simulink model "KUKA_AdaptiveComposite"  (R2021a)
settings: Solver=FixedStepAuto  StartTime=0.0  StopTime=2  FixedStep=0.001  RelTol=1e-3
InitFcn:
  | Gamma=eye(4)*0.1;
  | K=[1600 1600 1600 1600;80 80 80 80];
  | 
  | Gamma1=diag([20,10,10,15]);
  | K1=[1600 900 900 900;40 40 40 40];
  | 
  | Gamma2=eye(4)*5;
  | K2=[1600 900 900 900; 60 60 60 60];
values from neighbouring files (symbols this model uses):
  m = {0 0 0 0 0}    [DynMatrixCalculator.m]
  N = {zeros(3,1) zeros(3,1) zeros(3,1) zeros(3,1) zeros(3,1)}    [DynMatrixCalculator.m]
undefined symbols (not defined in the file or in its folder): X, Y, Z
libraries: nesl_utility x51, sm_lib x48
(part 1 of 4)
settings Model: Creator=Rahman Ardakanian  LastModifiedBy=hooma
settings SolverCC: AlgebraicLoopSolver=TrustRegion
settings DebuggingCC: SFMachineParentedDataDiag=warning  ArithmeticOperatorsInVariantConditions=warning
settings SFSimCC: CustomCodeUndefinedFunction=UseInterfaceOnly
settings CodeAppCC: StateflowObjectComments=on

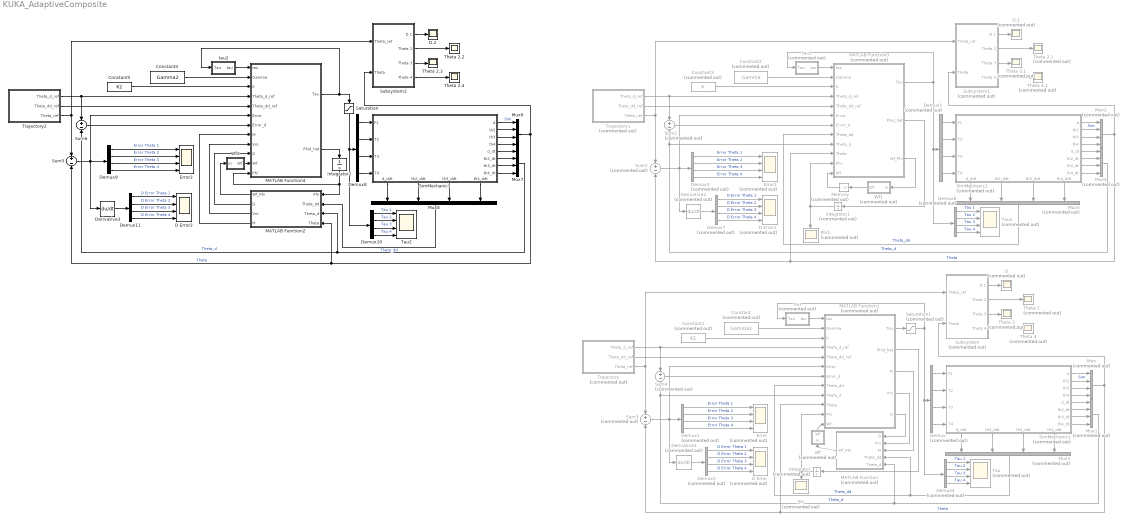
== system KUKA_AdaptiveComposite ==
  Constant : Constant  Commented=on  Value=Gamma1
  Constant1 : Constant  Commented=on  Value=K1
  Constant2 : Constant  Commented=on  Value=Gamma
  Constant3 : Constant  Commented=on  Value=K
  Constant4 : Constant  Value=Gamma2
  Constant5 : Constant  Value=K2
  D : Scope  Commented=on
  D Error : Scope  Commented=on  NumInputPorts=4
  D Error1 : Scope  Commented=on  NumInputPorts=4
  D Error2 : Scope  NumInputPorts=4
  D.1 : Scope  Commented=on
  D.2 : Scope
  Demux{,1..7} (8 alike) : Demux  Commented=on
  Demux{8..11} (4 alike) : Demux
  Derivative1 : Derivative  Commented=on
  Derivative2 : Derivative  Commented=on
  Derivative3 : Derivative
  Error : Scope  Commented=on  NumInputPorts=4
  Error1 : Scope  Commented=on  NumInputPorts=4
  Error2 : Scope  NumInputPorts=4
  Integrator : Integrator  Commented=on  InitialCondition=[17.65,7.84,10.64,8.58,0.186*0.8,0.082*0.8,0.176*0.8,0.166*0.8]
  Integrator1 : Integrator  Commented=on  InitialCondition=[17.65,7.84,10.64,8.58,0.186*0.8,0.082*0.8,0.176*0.8,0.166*0.8]
  Integrator2 : Integrator  InitialCondition=[17.65,7.84,10.64,8.58,0.186*0.8,0.082*0.8,0.176*0.8,0.166*0.8]
  MATLAB Function : MATLAB Function  Commented=on  TreatAsAtomicUnit=on
  MATLAB Function1 : MATLAB Function  Commented=on  TreatAsAtomicUnit=on
  MATLAB Function2 : MATLAB Function  TreatAsAtomicUnit=on
  MATLAB Function3 : MATLAB Function  Commented=on  TreatAsAtomicUnit=on
  MATLAB Function4 : MATLAB Function  TreatAsAtomicUnit=on
  Memory : Memory  Commented=on  InitialCondition=[1,1,1,1]'*0.001
  Mux{,1..5} (6 alike) : Mux  Commented=on
  Mux6 : Mux
  Mux7 : Mux
  Mux8 : Mux
  Phi : Scope  Commented=on
  Phi1 : Scope  Commented=on
  Saturation : Saturate  UpperLimit=[200, 100,100,100]  LowerLimit=-[200, 100,100,100]
  Saturation1 : Saturate  Commented=on  UpperLimit=[200,50,90,30]  LowerLimit=-[200,50,10,10]
  SimMechanic1 : Subsystem  Commented=on
      settings: PortSchema="{\"entries\":[{\"content\":{\"sides\":[{\"content\":{\"connectorIds\":[\"In1\",\"In2\",\"In3\",\"In4\"]},\"type\":\"ConnectorPlacement.EquallySpacedRectSide\",\"uuid\":\"b6277f71-9209-40f9-aaeb-b6c9fa71fb46\"},{\"content\":{\"connectorIds\":[\"Out1\",\"Out2\",\"Out3\",\"Out4\",\"Out5\",\"Out6\",\"Out7\",\"Out8\"],\"side\":\"RIGHT\"},\"type\":\"ConnectorPlacement.EquallySpacedRectSide\",\"uuid\":\"721928da-f16a-424c-b956-77fc0a07fccd\"},{\"content\":{\"connectorIds\":[],\"side\":\"TOP\"},\"type\":\"ConnectorPlacement.EquallySpacedRectSide\",\"uuid\":\"50ddb47d-7b49-4ba3-8344-b30f55dee798\"},{\"content\":{\"connectorIds\":[\"Out9\",\"Out10\",\"Out11\",\"Out12\"],\"side\":\"BOTTOM\"},\"type\":\"ConnectorPlacement.EquallySpacedRectSide\",\"uuid\":\"9af62a72-f078-4531-a2e0-d5b70f194bda\"}]},\"type\":\"ConnectorPlacement.EquallySpacedConnector\",\"uuid\":\"3abc4dda-09b7-4b6a-a507-303450cd9c4c\"}],\"packageUris\":[\"http://schema.mathworks.com/mf0/Connector/R2020b\"],\"version\":\"1.0\"}"
  SimMechanic2 : Subsystem  Commented=on
      settings: PortSchema="{\"entries\":[{\"content\":{\"sides\":[{\"content\":{\"connectorIds\":[\"In1\",\"In2\",\"In3\",\"In4\"]},\"type\":\"ConnectorPlacement.EquallySpacedRectSide\",\"uuid\":\"b6277f71-9209-40f9-aaeb-b6c9fa71fb46\"},{\"content\":{\"connectorIds\":[\"Out1\",\"Out2\",\"Out3\",\"Out4\",\"Out5\",\"Out6\",\"Out7\",\"Out8\"],\"side\":\"RIGHT\"},\"type\":\"ConnectorPlacement.EquallySpacedRectSide\",\"uuid\":\"721928da-f16a-424c-b956-77fc0a07fccd\"},{\"content\":{\"connectorIds\":[],\"side\":\"TOP\"},\"type\":\"ConnectorPlacement.EquallySpacedRectSide\",\"uuid\":\"50ddb47d-7b49-4ba3-8344-b30f55dee798\"},{\"content\":{\"connectorIds\":[\"Out9\",\"Out10\",\"Out11\",\"Out12\"],\"side\":\"BOTTOM\"},\"type\":\"ConnectorPlacement.EquallySpacedRectSide\",\"uuid\":\"9af62a72-f078-4531-a2e0-d5b70f194bda\"}]},\"type\":\"ConnectorPlacement.EquallySpacedConnector\",\"uuid\":\"3abc4dda-09b7-4b6a-a507-303450cd9c4c\"}],\"packageUris\":[\"http://schema.mathworks.com/mf0/Connector/R2020b\"],\"version\":\"1.0\"}"
  SimMechanic3 : Subsystem
      settings: PortSchema="{\"entries\":[{\"content\":{\"sides\":[{\"content\":{\"connectorIds\":[\"In1\",\"In2\",\"In3\",\"In4\"]},\"type\":\"ConnectorPlacement.EquallySpacedRectSide\",\"uuid\":\"b6277f71-9209-40f9-aaeb-b6c9fa71fb46\"},{\"content\":{\"connectorIds\":[\"Out1\",\"Out2\",\"Out3\",\"Out4\",\"Out5\",\"Out6\",\"Out7\",\"Out8\"],\"side\":\"RIGHT\"},\"type\":\"ConnectorPlacement.EquallySpacedRectSide\",\"uuid\":\"721928da-f16a-424c-b956-77fc0a07fccd\"},{\"content\":{\"connectorIds\":[],\"side\":\"TOP\"},\"type\":\"ConnectorPlacement.EquallySpacedRectSide\",\"uuid\":\"50ddb47d-7b49-4ba3-8344-b30f55dee798\"},{\"content\":{\"connectorIds\":[\"Out9\",\"Out10\",\"Out11\",\"Out12\"],\"side\":\"BOTTOM\"},\"type\":\"ConnectorPlacement.EquallySpacedRectSide\",\"uuid\":\"9af62a72-f078-4531-a2e0-d5b70f194bda\"}]},\"type\":\"ConnectorPlacement.EquallySpacedConnector\",\"uuid\":\"3abc4dda-09b7-4b6a-a507-303450cd9c4c\"}],\"packageUris\":[\"http://schema.mathworks.com/mf0/Connector/R2020b\"],\"version\":\"1.0\"}"
  Subsystem : Subsystem  Commented=on
  Subsystem1 : Subsystem  Commented=on
  Subsystem2 : Subsystem
  Sum{1..4} (4 alike) : Sum  Commented=on  Inputs=+|-
  Sum5 : Sum  Inputs=+|-
  Sum6 : Sum  Inputs=+|-
  Tau : Scope  Commented=on  NumInputPorts=4
  Tau1 : Scope  Commented=on  NumInputPorts=4
  Tau2 : Scope  NumInputPorts=4
  Theta 2 : Scope  Commented=on
  Theta 2.1 : Scope  Commented=on
  Theta 2.2 : Scope
  Theta 2.3 : Scope
  Theta 2.4 : Scope
  Theta 3 : Scope  Commented=on
  Theta 3.1 : Scope  Commented=on
  Theta 4 : Scope  Commented=on
  Theta 4.1 : Scope  Commented=on
  Trajectory : Subsystem  Commented=on
  Trajectory1 : Subsystem  Commented=on
  Trajectory2 : Subsystem
  Wf : Subsystem  Commented=on
  Wf1 : Subsystem  Commented=on
  Wf2 : Subsystem
  tau : Subsystem  Commented=on
  tau1 : Subsystem  Commented=on
  tau2 : Subsystem
  wires:
  Wf2/1(Wf) -> MATLAB Function4/11(Wf)
  Demux9/2 -> Error2/2  "Error Theta 2"
  Mux6/1 -> Subsystem2/2(Theta), Sum5/2, MATLAB Function2/4(Theta)  "Theta"
  Derivative3/1 -> Demux11/1
  Mux8/1 -> MATLAB Function2/2(Theta_dd)  "Theta_dd"
  SimMechanic3/1(d) -> Mux6/1  "Sim"
  SimMechanic3/2(th2) -> Mux6/2
  SimMechanic3/4(th4) -> Mux6/4
  Trajectory2/3(Theta_ref) -> Sum5/1, Subsystem2/1(Theta_ref)
  Demux8/3 -> SimMechanic3/3(T3)
  MATLAB Function2/1(Wf_Phi) -> Wf2/1(in)
  SimMechanic3/7(th3_dt) -> Mux7/3
  SimMechanic3/12(th4_ddt) -> Mux8/4
  Demux9/1 -> Error2/1  "Error Theta 1"
  SimMechanic3/3(th3) -> Mux6/3
  Demux10/2 -> Tau2/2  "Tau 2"
  Constant5/1 -> MATLAB Function4/3(K)
  Demux8/1 -> SimMechanic3/1(F1)
  SimMechanic3/8(th4_dt) -> Mux7/4
  SimMechanic3/5(d_dt) -> Mux7/1
  Demux9/3 -> Error2/3  "Error Theta 3"
  SimMechanic3/10(th2_ddt) -> Mux8/2
  Demux11/3 -> D Error2/3  "D Error Theta 3"
  SimMechanic3/6(th2_dt) -> Mux7/2
  SimMechanic3/11(th3_ddt) -> Mux8/3
  Demux11/4 -> D Error2/4  "D Error Theta 4"
  Trajectory2/1(Theta_d_ref) -> Sum6/1, MATLAB Function4/4(Theta_d_ref)
  Mux7/1 -> Sum6/2, MATLAB Function2/3(Theta_d)  "Theta_d"
  Trajectory2/2(Theta_dd_ref) -> MATLAB Function4/5(Theta_dd_ref)
  Demux10/3 -> Tau2/3  "Tau 3"
  Subsystem2/1(D 1) -> D.2/1
  Sum6/1 -> MATLAB Function4/7(Error_d)
  Demux11/2 -> D Error2/2  "D Error Theta 2"
  Subsystem2/4(Theta 4) -> Theta 2.4/1
  SimMechanic3/9(d_ddt) -> Mux8/1
  Demux10/1 -> Tau2/1  "Tau 1"
  Constant4/1 -> MATLAB Function4/2(Gamma)
  Subsystem2/2(Theta 2) -> Theta 2.2/1
  Subsystem2/3(Theta 3) -> Theta 2.3/1
  Demux10/4 -> Tau2/4  "Tau 4"
  Sum5/1 -> Derivative3/1, MATLAB Function4/6(Error), Demux9/1
  Demux8/4 -> SimMechanic3/4(T4)
  Demux11/1 -> D Error2/1  "D Error Theta 1"
  tau2/1(tau) -> MATLAB Function4/1(tau)
  Demux9/4 -> Error2/4  "Error Theta 4"
  Demux8/2 -> SimMechanic3/2(T2)
  MATLAB Function2/2(G) -> MATLAB Function4/10(G)
  MATLAB Function2/3(Vm) -> MATLAB Function4/9(Vm)
  MATLAB Function2/4(M) -> MATLAB Function4/8(M)
  MATLAB Function4/2(Phid_hat) -> Integrator2/1
  Integrator2/1 -> MATLAB Function2/1(Phi), MATLAB Function4/12(Phi)
  Saturation/1 -> Demux10/1, Demux8/1
  MATLAB Function4/1(Tau) -> tau2/1(Tau), Saturation/1
  Demux3/4 -> Error1/4  "Error Theta 4"
  Demux1/1 -> Error/1  "Error Theta 1"
  SimMechanic1/7(th3_dt) -> Mux1/3
  Trajectory/1(Theta_d_ref) -> Sum4/1, MATLAB Function1/4(Theta_d_ref)
  Demux5/4 -> D Error/4  "D Error Theta 4"
  Sum1/1 -> Derivative2/1, Demux3/1, MATLAB Function3/6(Error)
  SimMechanic2/7(th3_dt) -> Mux4/3
  SimMechanic1/12(th4_ddt) -> Mux3/4
  Demux/2 -> SimMechanic1/2(T2)
  Constant1/1 -> MATLAB Function1/3(K)
  Subsystem1/4(Theta 4) -> Theta 4.1/1
  Derivative1/1 -> Demux5/1
  SimMechanic1/6(th2_dt) -> Mux1/2
  SimMechanic2/4(th4) -> Mux2/4
  Demux/3 -> SimMechanic1/3(T3)
  Constant2/1 -> MATLAB Function3/2(Gamma)
  SimMechanic1/5(d_dt) -> Mux1/1
  Demux5/1 -> D Error/1  "D Error Theta 1"
  MATLAB Function1/4(Vm) -> MATLAB Function/2(Vm)
  Demux3/2 -> Error1/2  "Error Theta 2"
  tau/1(tau) -> MATLAB Function1/1(tau)
  MATLAB Function3/3(Wf_Phi) -> Wf1/1(in)
  Demux2/3 -> SimMechanic2/3(T3)
  SimMechanic1/1(d) -> Mux/1  "Sim"
  Integrator1/1 -> Phi1/1, MATLAB Function3/11(Phi)
  Demux6/2 -> Tau1/2  "Tau 2"
  Wf1/1(Wf) -> Memory/1
  Demux/1 -> SimMechanic1/1(F1)
  Subsystem/4(Theta 4) -> Theta 4/1
  SimMechanic1/11(th3_ddt) -> Mux3/3
  Saturation1/1 -> tau/1(Tau), Demux4/1, Demux/1
  MATLAB Function1/5(G) -> MATLAB Function/1(G)
  SimMechanic1/3(th3) -> Mux/3
  Demux3/1 -> Error1/1  "Error Theta 1"
  SimMechanic2/12(th4_ddt) -> Mux5/4
  SimMechanic2/3(th3) -> Mux2/3
  Memory/1 -> MATLAB Function3/12(Wf)
  Demux/4 -> SimMechanic1/4(T4)
  SimMechanic2/5(d_dt) -> Mux4/1
  Demux5/2 -> D Error/2  "D Error Theta 2"
  Demux4/3 -> Tau/3  "Tau 3"
  Subsystem/2(Theta 2) -> Theta 2/1
  Demux4/4 -> Tau/4  "Tau 4"
  Demux4/1 -> Tau/1  "Tau 1"
  Mux/1 -> Subsystem/2(Theta), MATLAB Function1/10(Theta), Sum3/2  "Theta"
  Demux1/3 -> Error/3  "Error Theta 3"
  Demux2/2 -> SimMechanic2/2(T2)
  SimMechanic1/2(th2) -> Mux/2
  Mux5/1 -> MATLAB Function3/8(Theta_dd)  "Theta_dd"
  Demux5/3 -> D Error/3  "D Error Theta 3"
  Demux6/1 -> Tau1/1  "Tau 1"
  Demux2/4 -> SimMechanic2/4(T4)
  Demux4/2 -> Tau/2  "Tau 2"
  SimMechanic1/8(th4_dt) -> Mux1/4
  SimMechanic1/10(th2_ddt) -> Mux3/2
  Subsystem/1(D 1) -> D/1
  Integrator/1 -> MATLAB Function1/11(Phi), Phi/1
  SimMechanic1/9(d_ddt) -> Mux3/1
  Mux3/1 -> MATLAB Function1/8(Theta_dd), MATLAB Function/4(Theta_dd)  "Theta_dd"
  Mux1/1 -> MATLAB Function/5(Theta_d), Sum4/2, MATLAB Function1/9(Theta_d)  "Theta_d"
  Sum4/1 -> MATLAB Function1/7(Error_d)
  Subsystem1/2(Theta 2) -> Theta 2.1/1
  Demux6/3 -> Tau1/3  "Tau 3"
  SimMechanic2/2(th2) -> Mux2/2
  Constant3/1 -> MATLAB Function3/3(K)
  Demux7/1 -> D Error1/1  "D Error Theta 1"
  SimMechanic1/4(th4) -> Mux/4
  Subsystem1/1(D 1) -> D.1/1
  Subsystem/3(Theta 3) -> Theta 3/1
  Demux6/4 -> Tau1/4  "Tau 4"
  Constant/1 -> MATLAB Function1/2(Gamma)
  Wf/1(Wf) -> MATLAB Function1/12(Wf)
  Demux1/2 -> Error/2  "Error Theta 2"
  MATLAB Function/1(Wf_Phi) -> Wf/1(in)
  SimMechanic2/1(d) -> Mux2/1  "Sim"
  MATLAB Function1/3(M) -> MATLAB Function/3(M)
  SimMechanic2/8(th4_dt) -> Mux4/4
  Trajectory/2(Theta_dd_ref) -> MATLAB Function1/5(Theta_dd_ref)
  SimMechanic2/9(d_ddt) -> Mux5/1
  Demux7/2 -> D Error1/2  "D Error Theta 2"
  MATLAB Function3/1(Tau) -> tau1/1(Tau), Demux6/1, Demux2/1
  MATLAB Function1/2(Phid_hat) -> Integrator/1
  SimMechanic2/11(th3_ddt) -> Mux5/3
  SimMechanic2/6(th2_dt) -> Mux4/2
  Derivative2/1 -> Demux7/1
  Mux2/1 -> Subsystem1/2(Theta), MATLAB Function3/10(Theta), Sum1/2  "Theta"
  Mux4/1 -> Sum2/2, MATLAB Function3/9(Theta_d)  "Theta_d"
  Sum3/1 -> Derivative1/1, Demux1/1, MATLAB Function1/6(Error)
  tau1/1(tau) -> MATLAB Function3/1(tau)
  MATLAB Function1/1(Tau) -> Saturation1/1
  MATLAB Function3/2(Phid_hat) -> Integrator1/1
  Demux3/3 -> Error1/3  "Error Theta 3"
  Demux2/1 -> SimMechanic2/1(F1)
  Trajectory1/2(Theta_dd_ref) -> MATLAB Function3/5(Theta_dd_ref)
  Trajectory/3(Theta_ref) -> Sum3/1, Subsystem/1(Theta_ref)
  Demux1/4 -> Error/4  "Error Theta 4"
  Trajectory1/1(Theta_d_ref) -> Sum2/1, MATLAB Function3/4(Theta_d_ref)
  SimMechanic2/10(th2_ddt) -> Mux5/2
  Demux7/4 -> D Error1/4  "D Error Theta 4"
  Sum2/1 -> MATLAB Function3/7(Error_d)
  Trajectory1/3(Theta_ref) -> Sum1/1, Subsystem1/1(Theta_ref)
  Subsystem1/3(Theta 3) -> Theta 3.1/1
  Demux7/3 -> D Error1/3  "D Error Theta 3"

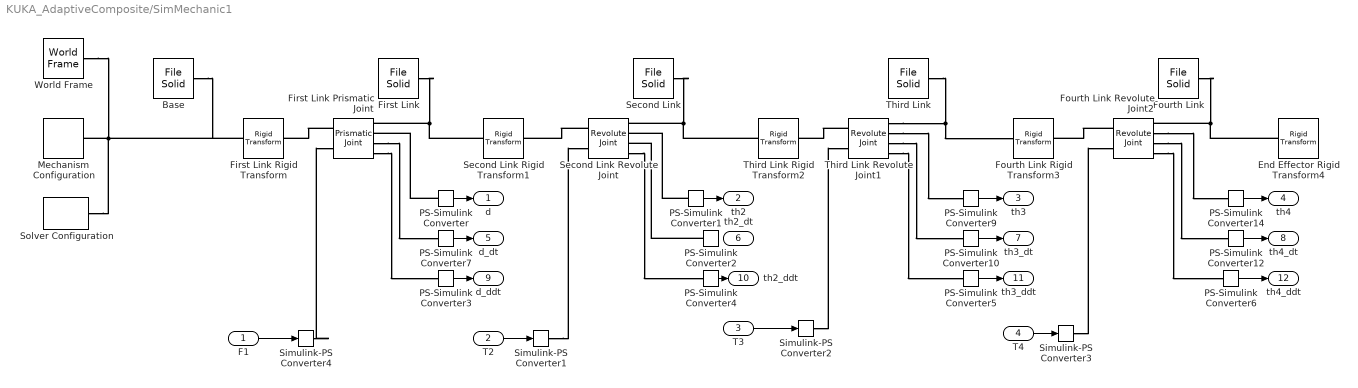
== system KUKA_AdaptiveComposite/SimMechanic1 ==
  F1 : Inport
  T2 : Inport  Port=2
  T3 : Inport  Port=3
  T4 : Inport  Port=4
  Base : sm_lib/Body Elements/File Solid  ExtGeomFileName=L0.STL  UnitType=Custom  ExtGeomFileUnits=mm  StepReaderType=HEX  ExportConvexHullGeometry=off  InertiaType=Custom  Mass=40.117  MassUnits=kg  CenterOfMass=[0 -0.033 0]  CenterOfMassUnits=m  MomentsOfInertia=[13.366 13.428 0.066]  MomentsOfInertiaUnits=kg*m^2  ProductsOfInertia=[0 0 0]  ProductsOfInertiaUnits=kg*m^2  BasedOnType=Density  Density=1000  DensityUnits=kg/m^3  DoExposeReferenceFrame=on  SerializedFrames=<Frames/>  GraphicType=FromGeometry  MarkerShape=Sphere  MarkerSize=10  GraphicVisPropType=SimpleVisualProperties  GraphicDiffuseColor=[0.5 0.5 0.5]  GraphicSpecularColor=[0.5 0.5 0.5 1.0]  GraphicAmbientColor=[0.15 0.15 0.15 1.0]  GraphicEmissiveColor=[0.0 0.0 0.0 1.0]  GraphicShininess=75  GraphicOpacity=1.0
  End Effector Rigid Transform4 : sm_lib/Frames and Transforms/Rigid Transform  TranslationMethod=Cartesian  TranslationStandardOffset=0  TranslationLengthUnit=mm  TranslationStandardAxis=+Z  TranslationCartesianOffset=[382.6 20 0]  TranslationROffset=0  TranslationROffsetUnits=m  TranslationZOffset=0  TranslationZOffsetUnits=m  TranslationThetaOffset=0  TranslationThetaOffsetUnits=deg  RotationMethod=AlignedAxes  RotationAngleUnits=deg  RotationStandardAxis=+Z  RotationAngle=0.0  RotationArbitraryAxis=[0 0 1]  FollAlignAxisA=+X  BaseAlignAxisA=+X  FollAlignAxisB=+Y  BaseAlignAxisB=+Y  RotationSequenceAxes=FollowerAxes  RotationSequence=XYX  RotationSequenceAngles=[0 0 0]  RotationSequenceAnglesUnits=deg  RotationMatrix=[1 0 0; 0 1 0; 0 0 1]
  First Link : sm_lib/Body Elements/File Solid  ExtGeomFileName=L1.STL  UnitType=Custom  ExtGeomFileUnits=mm  StepReaderType=HEX  ExportConvexHullGeometry=off  InertiaType=Custom  Mass=22.064  MassUnits=kg  CenterOfMass=[-0.031 0.094 0]  CenterOfMassUnits=m  MomentsOfInertia=[0.134 0.165 0.186]  MomentsOfInertiaUnits=kg*m^2  ProductsOfInertia=[0 0.001 -0.012]  ProductsOfInertiaUnits=kg*m^2  BasedOnType=Density  Density=1000  DensityUnits=kg/m^3  DoExposeReferenceFrame=on  SerializedFrames=<Frames/>  GraphicType=FromGeometry  MarkerShape=Sphere  MarkerSize=10  GraphicVisPropType=SimpleVisualProperties  GraphicDiffuseColor=[0.5 0.5 0.5]  GraphicSpecularColor=[0.5 0.5 0.5 1.0]  GraphicAmbientColor=[0.15 0.15 0.15 1.0]  GraphicEmissiveColor=[0.0 0.0 0.0 1.0]  GraphicShininess=75  GraphicOpacity=1.0
  First Link Prismatic Joint : sm_lib/Joints/Prismatic Joint  JointMode=Normal  SenseConstraintForce=off  SenseConstraintForceX=off  SenseConstraintForceY=off  SenseConstraintForceZ=off  SenseConstraintTorque=off  SenseConstraintTorqueX=off  SenseConstraintTorqueY=off  SenseConstraintTorqueZ=off  SenseTotalForce=off  SenseTotalForceX=off  SenseTotalForceY=off  SenseTotalForceZ=off  SenseTotalTorque=off  SenseTotalTorqueX=off  SenseTotalTorqueY=off  SenseTotalTorqueZ=off  CompositeWrenchDir=FollowerOnBase  CompositeWrenchFrame=BaseFrame  EquilibriumPosition=0  EquilibriumPositionUnits=m  SpringStiffness=0  SpringStiffnessUnits=N/m  DampingCoefficient=0  DampingCoefficientUnits=N/(m/s)  TorqueActuationMode=InputTorque  MotionActuationMode=ComputedMotion  SensePosition=on  SenseVelocity=on  SenseAcceleration=on  SenseTorqueForce=off  SenseLowerLimitTorqueForce=off  SenseUpperLimitTorqueForce=off  LowerLimitSpecify=off  LowerLimitBound=-1  LowerLimitBoundUnits=m  LowerLimitStiffness=1e6  LowerLimitStiffnessUnits=N/m  LowerLimitDamping=1e3  LowerLimitDampingUnits=N/(m/s)  LowerLimitTransitionRegionWidth=1e-4  LowerLimitTransitionRegionWidthUnits=m  UpperLimitSpecify=off  UpperLimitBound=1  UpperLimitBoundUnits=m  UpperLimitStiffness=1e6  UpperLimitStiffnessUnits=N/m  UpperLimitDamping=1e3  UpperLimitDampingUnits=N/(m/s)  UpperLimitTransitionRegionWidth=1e-4  UpperLimitTransitionRegionWidthUnits=m  PositionTargetSpecify=off  PositionTargetPriority=High  PositionTargetValue=0  PositionTargetValueUnits=m  VelocityTargetSpecify=off  VelocityTargetPriority=High  VelocityTargetValue=0  VelocityTargetValueUnits=m/s
  First Link Rigid Transform : sm_lib/Frames and Transforms/Rigid Transform  TranslationMethod=Cartesian  TranslationStandardOffset=0  TranslationLengthUnit=mm  TranslationStandardAxis=+Z  TranslationCartesianOffset=[0 0 0]  TranslationROffset=0  TranslationROffsetUnits=m  TranslationZOffset=0  TranslationZOffsetUnits=m  TranslationThetaOffset=0  TranslationThetaOffsetUnits=deg  RotationMethod=AlignedAxes  RotationAngleUnits=deg  RotationStandardAxis=+Z  RotationAngle=0.0  RotationArbitraryAxis=[0 0 1]  FollAlignAxisA=+X  BaseAlignAxisA=+X  FollAlignAxisB=+Y  BaseAlignAxisB=+Y  RotationSequenceAxes=FollowerAxes  RotationSequence=XYX  RotationSequenceAngles=[0 0 0]  RotationSequenceAnglesUnits=deg  RotationMatrix=[1 0 0; 0 1 0; 0 0 1]
  Fourth Link : sm_lib/Body Elements/File Solid  ExtGeomFileName=L4.STL  UnitType=Custom  ExtGeomFileUnits=mm  StepReaderType=HEX  ExportConvexHullGeometry=off  InertiaType=Custom  Mass=10.723  MassUnits=kg  CenterOfMass=[0.143 0.015 -0.001]  CenterOfMassUnits=m  MomentsOfInertia=[0.018 0.166 0.164]  MomentsOfInertiaUnits=kg*m^2  ProductsOfInertia=[0 -0.001 0.009]  ProductsOfInertiaUnits=kg*m^2  BasedOnType=Density  Density=1000  DensityUnits=kg/m^3  DoExposeReferenceFrame=on  SerializedFrames=<Frames/>  GraphicType=FromGeometry  MarkerShape=Sphere  MarkerSize=10  GraphicVisPropType=SimpleVisualProperties  GraphicDiffuseColor=[0.5 0.5 0.5]  GraphicSpecularColor=[0.5 0.5 0.5 1.0]  GraphicAmbientColor=[0.15 0.15 0.15 1.0]  GraphicEmissiveColor=[0.0 0.0 0.0 1.0]  GraphicShininess=75  GraphicOpacity=1.0
  Fourth Link Revolute Joint2 : sm_lib/Joints/Revolute Joint  JointMode=Normal  SenseConstraintForce=off  SenseConstraintForceX=off  SenseConstraintForceY=off  SenseConstraintForceZ=off  SenseConstraintTorque=off  SenseConstraintTorqueX=off  SenseConstraintTorqueY=off  SenseConstraintTorqueZ=off  SenseTotalForce=off  SenseTotalForceX=off  SenseTotalForceY=off  SenseTotalForceZ=off  SenseTotalTorque=off  SenseTotalTorqueX=off  SenseTotalTorqueY=off  SenseTotalTorqueZ=off  CompositeWrenchDir=FollowerOnBase  CompositeWrenchFrame=BaseFrame  EquilibriumPosition=0  EquilibriumPositionUnits=deg  SpringStiffness=0  SpringStiffnessUnits=N*m/deg  DampingCoefficient=0  DampingCoefficientUnits=N*m/(deg/s)  TorqueActuationMode=InputTorque  MotionActuationMode=ComputedMotion  SensePosition=on  SenseVelocity=on  SenseAcceleration=on  SenseTorqueForce=off  SenseLowerLimitTorqueForce=off  SenseUpperLimitTorqueForce=off  LowerLimitSpecify=off  LowerLimitBound=-90  LowerLimitBoundUnits=deg  LowerLimitStiffness=1e4  LowerLimitStiffnessUnits=N*m/deg  LowerLimitDamping=10  LowerLimitDampingUnits=N*m/(deg/s)  LowerLimitTransitionRegionWidth=0.1  LowerLimitTransitionRegionWidthUnits=deg  UpperLimitSpecify=off  UpperLimitBound=90  UpperLimitBoundUnits=deg  UpperLimitStiffness=1e4  UpperLimitStiffnessUnits=N*m/deg  UpperLimitDamping=10  UpperLimitDampingUnits=N*m/(deg/s)  UpperLimitTransitionRegionWidth=0.1  UpperLimitTransitionRegionWidthUnits=deg  PositionTargetSpecify=off  PositionTargetPriority=High  PositionTargetValue=0  PositionTargetValueUnits=deg  VelocityTargetSpecify=off  VelocityTargetPriority=High  VelocityTargetValue=0  VelocityTargetValueUnits=deg/s
  Fourth Link Rigid Transform3 : sm_lib/Frames and Transforms/Rigid Transform  TranslationMethod=Cartesian  TranslationStandardOffset=0  TranslationLengthUnit=mm  TranslationStandardAxis=+Z  TranslationCartesianOffset=[290 0 0]  TranslationROffset=0  TranslationROffsetUnits=m  TranslationZOffset=0  TranslationZOffsetUnits=m  TranslationThetaOffset=0  TranslationThetaOffsetUnits=deg  RotationMethod=AlignedAxes  RotationAngleUnits=deg  RotationStandardAxis=+Z  RotationAngle=0.0  RotationArbitraryAxis=[0 0 1]  FollAlignAxisA=+X  BaseAlignAxisA=-Y  FollAlignAxisB=+Z  BaseAlignAxisB=+Z  RotationSequenceAxes=FollowerAxes  RotationSequence=XYX  RotationSequenceAngles=[0 0 0]  RotationSequenceAnglesUnits=deg  RotationMatrix=[1 0 0; 0 1 0; 0 0 1]
  Mechanism Configuration : sm_lib/Utilities/Mechanism Configuration  UniformGravity=Constant  GravityVector=[0 -9.80665 0]  GravityVectorUnits=m/s^2  GravityUnits=m/s^2  LinearizationDelta=0.001  JointModeTransitionNonlinearIterations=2
  PS-Simulink Converter : nesl_utility/PS-Simulink Converter  PhysicalDomain=network_engine_domain  SubClassName=ps_output  LeftPortType=input  RightPortType=output  PseudoPeriodic=off  Frequencies=[]  Unit=m  AffineConversion=off
      settings: SourceProductBaseCode=PW,SS
  PS-Simulink Converter1 : nesl_utility/PS-Simulink Converter  PhysicalDomain=network_engine_domain  SubClassName=ps_output  LeftPortType=input  RightPortType=output  PseudoPeriodic=off  Frequencies=[]  Unit=rad  AffineConversion=off
      settings: SourceProductBaseCode=PW,SS
  PS-Simulink Converter10 : nesl_utility/PS-Simulink Converter  PhysicalDomain=network_engine_domain  SubClassName=ps_output  LeftPortType=input  RightPortType=output  PseudoPeriodic=off  Frequencies=[]  Unit=rad/s  AffineConversion=off
      settings: SourceProductBaseCode=PW,SS
  PS-Simulink Converter12 : nesl_utility/PS-Simulink Converter  PhysicalDomain=network_engine_domain  SubClassName=ps_output  LeftPortType=input  RightPortType=output  PseudoPeriodic=off  Frequencies=[]  Unit=rad/s  AffineConversion=off
      settings: SourceProductBaseCode=PW,SS
  PS-Simulink Converter14 : nesl_utility/PS-Simulink Converter  PhysicalDomain=network_engine_domain  SubClassName=ps_output  LeftPortType=input  RightPortType=output  PseudoPeriodic=off  Frequencies=[]  Unit=rad  AffineConversion=off
      settings: SourceProductBaseCode=PW,SS
  PS-Simulink Converter2 : nesl_utility/PS-Simulink Converter  PhysicalDomain=network_engine_domain  SubClassName=ps_output  LeftPortType=input  RightPortType=output  PseudoPeriodic=off  Frequencies=[]  Unit=rad/s  AffineConversion=off
      settings: SourceProductBaseCode=PW,SS
  PS-Simulink Converter3 : nesl_utility/PS-Simulink Converter  PhysicalDomain=network_engine_domain  SubClassName=ps_output  LeftPortType=input  RightPortType=output  PseudoPeriodic=off  Frequencies=[]  Unit=m/s^2  AffineConversion=off
      settings: SourceProductBaseCode=PW,SS
  PS-Simulink Converter4 : nesl_utility/PS-Simulink Converter  PhysicalDomain=network_engine_domain  SubClassName=ps_output  LeftPortType=input  RightPortType=output  PseudoPeriodic=off  Frequencies=[]  Unit=rad/s^2  AffineConversion=off
      settings: SourceProductBaseCode=PW,SS
  PS-Simulink Converter5 : nesl_utility/PS-Simulink Converter  PhysicalDomain=network_engine_domain  SubClassName=ps_output  LeftPortType=input  RightPortType=output  PseudoPeriodic=off  Frequencies=[]  Unit=rad/s^2  AffineConversion=off
      settings: SourceProductBaseCode=PW,SS
  PS-Simulink Converter6 : nesl_utility/PS-Simulink Converter  PhysicalDomain=network_engine_domain  SubClassName=ps_output  LeftPortType=input  RightPortType=output  PseudoPeriodic=off  Frequencies=[]  Unit=rad/s^2  AffineConversion=off
      settings: SourceProductBaseCode=PW,SS
  PS-Simulink Converter7 : nesl_utility/PS-Simulink Converter  PhysicalDomain=network_engine_domain  SubClassName=ps_output  LeftPortType=input  RightPortType=output  PseudoPeriodic=off  Frequencies=[]  Unit=m/s  AffineConversion=off
      settings: SourceProductBaseCode=PW,SS
  PS-Simulink Converter9 : nesl_utility/PS-Simulink Converter  PhysicalDomain=network_engine_domain  SubClassName=ps_output  LeftPortType=input  RightPortType=output  PseudoPeriodic=off  Frequencies=[]  Unit=rad  AffineConversion=off
      settings: SourceProductBaseCode=PW,SS
  Second Link : sm_lib/Body Elements/File Solid  ExtGeomFileName=L2.STL  UnitType=Custom  ExtGeomFileUnits=mm  StepReaderType=HEX  ExportConvexHullGeometry=off  InertiaType=Custom  Mass=9.805  MassUnits=kg  CenterOfMass=[-0.005 -0.001 0.082]  CenterOfMassUnits=m  MomentsOfInertia=[0.082 0.053 0.058]  MomentsOfInertiaUnits=kg*m^2  ProductsOfInertia=[-0.001 0 0]  ProductsOfInertiaUnits=kg*m^2  BasedOnType=Density  Density=1000  DensityUnits=kg/m^3  DoExposeReferenceFrame=on  SerializedFrames=<Frames/>  GraphicType=FromGeometry  MarkerShape=Sphere  MarkerSize=10  GraphicVisPropType=SimpleVisualProperties  GraphicDiffuseColor=[0.5 0.5 0.5]  GraphicSpecularColor=[0.5 0.5 0.5 1.0]  GraphicAmbientColor=[0.15 0.15 0.15 1.0]  GraphicEmissiveColor=[0.0 0.0 0.0 1.0]  GraphicShininess=75  GraphicOpacity=1.0
  Second Link Revolute Joint : sm_lib/Joints/Revolute Joint  JointMode=Normal  SenseConstraintForce=off  SenseConstraintForceX=off  SenseConstraintForceY=off  SenseConstraintForceZ=off  SenseConstraintTorque=off  SenseConstraintTorqueX=off  SenseConstraintTorqueY=off  SenseConstraintTorqueZ=off  SenseTotalForce=off  SenseTotalForceX=off  SenseTotalForceY=off  SenseTotalForceZ=off  SenseTotalTorque=off  SenseTotalTorqueX=off  SenseTotalTorqueY=off  SenseTotalTorqueZ=off  CompositeWrenchDir=FollowerOnBase  CompositeWrenchFrame=BaseFrame  EquilibriumPosition=0  EquilibriumPositionUnits=deg  SpringStiffness=0  SpringStiffnessUnits=N*m/deg  DampingCoefficient=0  DampingCoefficientUnits=N*m/(deg/s)  TorqueActuationMode=InputTorque  MotionActuationMode=ComputedMotion  SensePosition=on  SenseVelocity=on  SenseAcceleration=on  SenseTorqueForce=off  SenseLowerLimitTorqueForce=off  SenseUpperLimitTorqueForce=off  LowerLimitSpecify=off  LowerLimitBound=-90  LowerLimitBoundUnits=deg  LowerLimitStiffness=1e4  LowerLimitStiffnessUnits=N*m/deg  LowerLimitDamping=10  LowerLimitDampingUnits=N*m/(deg/s)  LowerLimitTransitionRegionWidth=0.1  LowerLimitTransitionRegionWidthUnits=deg  UpperLimitSpecify=off  UpperLimitBound=90  UpperLimitBoundUnits=deg  UpperLimitStiffness=1e4  UpperLimitStiffnessUnits=N*m/deg  UpperLimitDamping=10  UpperLimitDampingUnits=N*m/(deg/s)  UpperLimitTransitionRegionWidth=0.1  UpperLimitTransitionRegionWidthUnits=deg  PositionTargetSpecify=off  PositionTargetPriority=High  PositionTargetValue=0  PositionTargetValueUnits=deg  VelocityTargetSpecify=off  VelocityTargetPriority=High  VelocityTargetValue=0  VelocityTargetValueUnits=deg/s
  Second Link Rigid Transform1 : sm_lib/Frames and Transforms/Rigid Transform  TranslationMethod=Cartesian  TranslationStandardOffset=0  TranslationLengthUnit=mm  TranslationStandardAxis=+Z  TranslationCartesianOffset=[0 197 0]  TranslationROffset=0  TranslationROffsetUnits=m  TranslationZOffset=0  TranslationZOffsetUnits=m  TranslationThetaOffset=0  TranslationThetaOffsetUnits=deg  RotationMethod=AlignedAxes  RotationAngleUnits=deg  RotationStandardAxis=+Z  RotationAngle=0.0  RotationArbitraryAxis=[0 0 1]  FollAlignAxisA=+X  BaseAlignAxisA=+X  FollAlignAxisB=+Y  BaseAlignAxisB=-Z  RotationSequenceAxes=FollowerAxes  RotationSequence=XYX  RotationSequenceAngles=[0 0 0]  RotationSequenceAnglesUnits=deg  RotationMatrix=[1 0 0; 0 1 0; 0 0 1]
  Simulink-PS Converter{1..4} (4 alike) : nesl_utility/Simulink-PS Converter  PhysicalDomain=network_engine_domain  SubClassName=ps_input  LeftPortType=input  RightPortType=output  PseudoPeriodic=off  Frequencies=[]  NoiseDistribution=none  NoiseParameters=[]  Unit=1  AffineConversion=off  FilteringAndDerivatives=provide  SimscapeFilterOrder=1  InputFilterTimeConstant=0.001  UdotUserProvided=0
      settings: SourceProductBaseCode=PW,SS
  Solver Configuration : nesl_utility/Solver Configuration  PhysicalDomain=network_engine_domain  SubClassName=solver  LeftPortType=input  RightPortType=generic  Tones=[]  Harmonics=[]  SimulateNoise=off  Profile=off  UseLocalSampling=off  EnableSwitchedLinearOptims=on  FrequencyDomain=off  UseCCode=off  RelTol=0.001  AbsTol=1e-06  MinStep=1e-09  ToWorkspace=off  RevertToSquareIcSolve=off  NumHomotopyIterations=100  PhasorMode=off  PhasorModeNumHarmonics=1  DoDC=off  ResidualTolerance=1e-09  UseLocalSolver=off  LocalSolverChoice=NE_BACKWARD_EULER_ADVANCER  LocalSolverSampleTime=0.001  DoFixedCost=off  MaxNonlinIter=3  MaxModeIter=2  ComputeImpulses=off  ImpulseIterations=2  LinearAlgebra=Sparse  EquationFormulation=NE_TIME_EF  DelaysMemoryBudget=1024  AutomaticFiltering=on  FilteringTimeConstant=0.001  PartitionStorageMethod=AS_NEEDED  PartitionMemoryBudget=1024  PartitionMethod=FAST
      settings: SourceProductBaseCode=PW,SS
  Third Link : sm_lib/Body Elements/File Solid  ExtGeomFileName=L3.STL  UnitType=Custom  ExtGeomFileUnits=mm  StepReaderType=HEX  ExportConvexHullGeometry=off  InertiaType=Custom  Mass=13.302  MassUnits=kg  CenterOfMass=[0.118 0.011 -0.001]  CenterOfMassUnits=m  MomentsOfInertia=[0.048 0.176 0.154]  MomentsOfInertiaUnits=kg*m^2  ProductsOfInertia=[0 0.002 0.003]  ProductsOfInertiaUnits=kg*m^2  BasedOnType=Density  Density=1000  DensityUnits=kg/m^3  DoExposeReferenceFrame=on  SerializedFrames=<Frames/>  GraphicType=FromGeometry  MarkerShape=Sphere  MarkerSize=10  GraphicVisPropType=SimpleVisualProperties  GraphicDiffuseColor=[0.5 0.5 0.5]  GraphicSpecularColor=[0.5 0.5 0.5 1.0]  GraphicAmbientColor=[0.15 0.15 0.15 1.0]  GraphicEmissiveColor=[0.0 0.0 0.0 1.0]  GraphicShininess=75  GraphicOpacity=1.0
  Third Link Revolute Joint1 : sm_lib/Joints/Revolute Joint  JointMode=Normal  SenseConstraintForce=off  SenseConstraintForceX=off  SenseConstraintForceY=off  SenseConstraintForceZ=off  SenseConstraintTorque=off  SenseConstraintTorqueX=off  SenseConstraintTorqueY=off  SenseConstraintTorqueZ=off  SenseTotalForce=off  SenseTotalForceX=off  SenseTotalForceY=off  SenseTotalForceZ=off  SenseTotalTorque=off  SenseTotalTorqueX=off  SenseTotalTorqueY=off  SenseTotalTorqueZ=off  CompositeWrenchDir=FollowerOnBase  CompositeWrenchFrame=BaseFrame  EquilibriumPosition=0  EquilibriumPositionUnits=deg  SpringStiffness=0  SpringStiffnessUnits=N*m/deg  DampingCoefficient=0  DampingCoefficientUnits=N*m/(deg/s)  TorqueActuationMode=InputTorque  MotionActuationMode=ComputedMotion  SensePosition=on  SenseVelocity=on  SenseAcceleration=on  SenseTorqueForce=off  SenseLowerLimitTorqueForce=off  SenseUpperLimitTorqueForce=off  LowerLimitSpecify=off  LowerLimitBound=-90  LowerLimitBoundUnits=deg  LowerLimitStiffness=1e4  LowerLimitStiffnessUnits=N*m/deg  LowerLimitDamping=10  LowerLimitDampingUnits=N*m/(deg/s)  LowerLimitTransitionRegionWidth=0.1  LowerLimitTransitionRegionWidthUnits=deg  UpperLimitSpecify=off  UpperLimitBound=90  UpperLimitBoundUnits=deg  UpperLimitStiffness=1e4  UpperLimitStiffnessUnits=N*m/deg  UpperLimitDamping=10  UpperLimitDampingUnits=N*m/(deg/s)  UpperLimitTransitionRegionWidth=0.1  UpperLimitTransitionRegionWidthUnits=deg  PositionTargetSpecify=off  PositionTargetPriority=High  PositionTargetValue=0  PositionTargetValueUnits=deg  VelocityTargetSpecify=off  VelocityTargetPriority=High  VelocityTargetValue=0  VelocityTargetValueUnits=deg/s
  Third Link Rigid Transform2 : sm_lib/Frames and Transforms/Rigid Transform  TranslationMethod=Cartesian  TranslationStandardOffset=0  TranslationLengthUnit=mm  TranslationStandardAxis=+Z  TranslationCartesianOffset=[0 0 152.5]  TranslationROffset=0  TranslationROffsetUnits=m  TranslationZOffset=0  TranslationZOffsetUnits=m  TranslationThetaOffset=0  TranslationThetaOffsetUnits=deg  RotationMethod=AlignedAxes  RotationAngleUnits=deg  RotationStandardAxis=+Z  RotationAngle=0.0  RotationArbitraryAxis=[0 0 1]  FollAlignAxisA=+X  BaseAlignAxisA=+Z  FollAlignAxisB=+Z  BaseAlignAxisB=-Y  RotationSequenceAxes=FollowerAxes  RotationSequence=XYX  RotationSequenceAngles=[0 0 0]  RotationSequenceAnglesUnits=deg  RotationMatrix=[1 0 0; 0 1 0; 0 0 1]
  World Frame : sm_lib/Frames and Transforms/World Frame
  d : Outport  VectorParamsAs1DForOutWhenUnconnected=off
  th2 : Outport  Port=2  VectorParamsAs1DForOutWhenUnconnected=off
  th3 : Outport  Port=3  VectorParamsAs1DForOutWhenUnconnected=off
  th4 : Outport  Port=4  VectorParamsAs1DForOutWhenUnconnected=off
  d_dt : Outport  Port=5  VectorParamsAs1DForOutWhenUnconnected=off
  th2_dt : Outport  Port=6  VectorParamsAs1DForOutWhenUnconnected=off
  th3_dt : Outport  Port=7  VectorParamsAs1DForOutWhenUnconnected=off
  th4_dt : Outport  Port=8  VectorParamsAs1DForOutWhenUnconnected=off
  d_ddt : Outport  Port=9
  th2_ddt : Outport  Port=10
  th3_ddt : Outport  Port=11
  th4_ddt : Outport  Port=12
  wires:
  F1/1 -> Simulink-PS Converter4/1
  PS-Simulink Converter/1 -> d/1
  T2/1 -> Simulink-PS Converter1/1
  PS-Simulink Converter9/1 -> th3/1
  PS-Simulink Converter14/1 -> th4/1
  PS-Simulink Converter7/1 -> d_dt/1
  PS-Simulink Converter10/1 -> th3_dt/1
  T3/1 -> Simulink-PS Converter2/1
  PS-Simulink Converter12/1 -> th4_dt/1
  T4/1 -> Simulink-PS Converter3/1
  PS-Simulink Converter1/1 -> th2/1
  PS-Simulink Converter3/1 -> d_ddt/1
  PS-Simulink Converter4/1 -> th2_ddt/1
  PS-Simulink Converter6/1 -> th4_ddt/1
  PS-Simulink Converter5/1 -> th3_ddt/1
  connections:
  End Effector Rigid Transform4/LConn1 -- Fourth Link/RConn1 -- Fourth Link Revolute Joint2/RConn1
  Third Link Rigid Transform2/LConn1 -- Second Link/RConn1 -- Second Link Revolute Joint/RConn1
  Solver Configuration/RConn1 -- World Frame/RConn1 -- First Link Rigid Transform/LConn1 -- Base/RConn1 -- Mechanism Configuration/RConn1
  Third Link Revolute Joint1/RConn1 -- Third Link/RConn1 -- Fourth Link Rigid Transform3/LConn1
  First Link Prismatic Joint/LConn1 -- First Link Rigid Transform/RConn1
  Fourth Link Revolute Joint2/LConn1 -- Fourth Link Rigid Transform3/RConn1
  Second Link Rigid Transform1/LConn1 -- First Link/RConn1 -- First Link Prismatic Joint/RConn1
  Third Link Revolute Joint1/LConn1 -- Third Link Rigid Transform2/RConn1
  Second Link Revolute Joint/LConn1 -- Second Link Rigid Transform1/RConn1
  Simulink-PS Converter4/RConn1 -- First Link Prismatic Joint/LConn2
  PS-Simulink Converter/LConn1 -- First Link Prismatic Joint/RConn2
  PS-Simulink Converter1/LConn1 -- Second Link Revolute Joint/RConn2
  Simulink-PS Converter1/RConn1 -- Second Link Revolute Joint/LConn2
  Simulink-PS Converter2/RConn1 -- Third Link Revolute Joint1/LConn2
  Simulink-PS Converter3/RConn1 -- Fourth Link Revolute Joint2/LConn2
  First Link Prismatic Joint/RConn3 -- PS-Simulink Converter7/LConn1
  PS-Simulink Converter2/LConn1 -- Second Link Revolute Joint/RConn3
  Third Link Revolute Joint1/RConn2 -- PS-Simulink Converter9/LConn1
  Third Link Revolute Joint1/RConn3 -- PS-Simulink Converter10/LConn1
  Fourth Link Revolute Joint2/RConn2 -- PS-Simulink Converter14/LConn1
  Fourth Link Revolute Joint2/RConn3 -- PS-Simulink Converter12/LConn1
  Fourth Link Revolute Joint2/RConn4 -- PS-Simulink Converter6/LConn1
  Third Link Revolute Joint1/RConn4 -- PS-Simulink Converter5/LConn1
  Second Link Revolute Joint/RConn4 -- PS-Simulink Converter4/LConn1
  First Link Prismatic Joint/RConn4 -- PS-Simulink Converter3/LConn1
